simulink model "dynamicsSimulink"  (R2018a)
settings: Solver=VariableStepAuto  StartTime=0.0  StopTime=10.0  RelTol=1e-3
libraries: vehdynlibtire x4
settings Model: Creator=Raval  LastModifiedBy=Raval

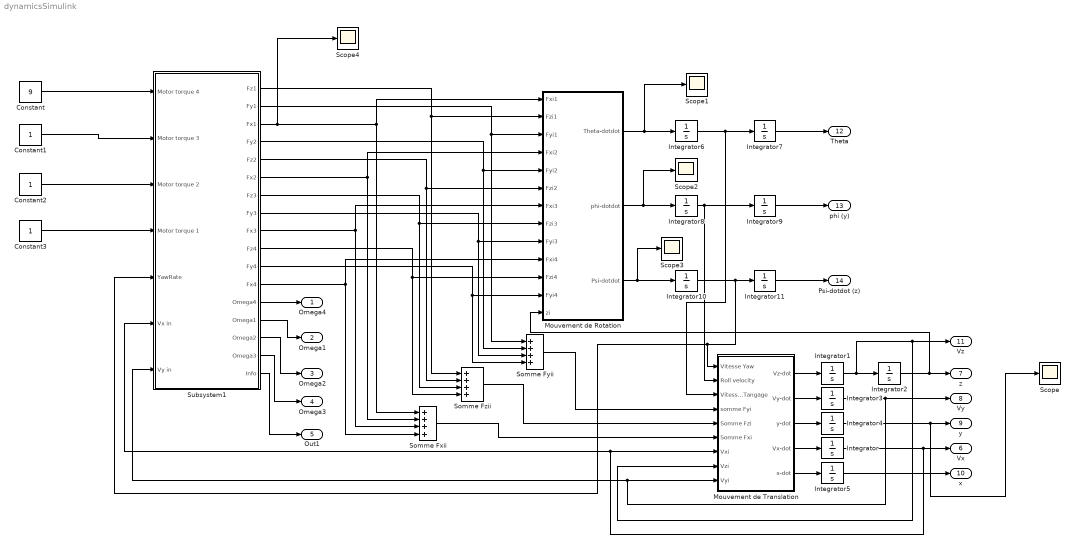
== system dynamicsSimulink ==
  Constant : Constant  Value=9
  Constant1 : Constant
  Constant2 : Constant
  Constant3 : Constant
  Integrator{,1..11} (12 alike) : Integrator
  Mouvement de Rotation : Subsystem
  Mouvement de Translation : Subsystem
  Scope{,1..4} (5 alike) : Scope
  Somme Fxii : Sum  Inputs=++++
  Somme Fyii : Sum  Inputs=++++
  Somme Fzii : Sum  Inputs=++++
  Subsystem1 : Subsystem
  Omega4 : Outport
  Omega1 : Outport  Port=2
  Omega2 : Outport  Port=3
  Omega3 : Outport  Port=4
  Out1 : Outport  Port=5
  Vx : Outport  Port=6
  z : Outport  Port=7
  Vy : Outport  Port=8
  y : Outport  Port=9
  x : Outport  Port=10
  Vz : Outport  Port=11
  Theta : Outport  Port=12
  phi (y) : Outport  Port=13
  Psi-dotdot (z) : Outport  Port=14
  wires:
  Integrator8/1 -> Mouvement de Translation/2(Roll velocity), Integrator9/1
  Integrator6/1 -> Mouvement de Translation/3(Vitesse Tangage), Integrator7/1
  Somme Fyii/1 -> Mouvement de Translation/4(somme Fyi)
  Somme Fzii/1 -> Mouvement de Translation/5(Somme Fzi)
  Somme Fxii/1 -> Mouvement de Translation/6(Somme Fxi)
  Integrator1/1 -> Mouvement de Translation/8(Vzi), Vz/1, Integrator2/1
  Mouvement de Translation/1(Vz-dot) -> Integrator1/1
  Mouvement de Translation/2(Vy-dot) -> Integrator3/1
  Mouvement de Translation/3(y-dot) -> Integrator4/1
  Mouvement de Translation/5(x-dot) -> Integrator5/1
  Subsystem1/3(Fx1) -> Scope4/1, Somme Fxii/1, Mouvement de Rotation/1(Fxi1)
  Subsystem1/1(Fz1) -> Mouvement de Rotation/2(Fzi1), Somme Fzii/1
  Subsystem1/2(Fy1) -> Mouvement de Rotation/3(Fyi1), Somme Fyii/1
  Subsystem1/6(Fx2) -> Somme Fxii/2, Mouvement de Rotation/4(Fxi2)
  Subsystem1/4(Fy2) -> Mouvement de Rotation/5(Fyi2), Somme Fyii/2
  Subsystem1/5(Fz2) -> Somme Fzii/2, Mouvement de Rotation/6(Fzi2)
  Subsystem1/9(Fx3) -> Mouvement de Rotation/7(Fxi3), Somme Fxii/3
  Subsystem1/7(Fz3) -> Somme Fzii/3, Mouvement de Rotation/8(Fzi3)
  Subsystem1/8(Fy3) -> Mouvement de Rotation/9(Fyi3), Somme Fyii/3
  Subsystem1/12(Fx4) -> Somme Fxii/4, Mouvement de Rotation/10(Fxi4)
  Subsystem1/10(Fz4) -> Somme Fzii/4, Mouvement de Rotation/11(Fzi4)
  Subsystem1/11(Fy4) -> Somme Fyii/4, Mouvement de Rotation/12(Fyi4)
  Integrator2/1 -> Mouvement de Rotation/13(zi), z/1
  Mouvement de Rotation/1(Theta-dotdot) -> Scope1/1, Integrator6/1
  Mouvement de Rotation/2(phi-dotdot) -> Scope2/1, Integrator8/1
  Mouvement de Rotation/3(Psi-dotdot) -> Scope3/1, Integrator10/1
  Constant/1 -> Subsystem1/1(Motor torque 4)
  Constant1/1 -> Subsystem1/2(Motor torque 3)
  Constant2/1 -> Subsystem1/3(Motor torque 2)
  Constant3/1 -> Subsystem1/4(Motor torque 1)
  Integrator10/1 -> Mouvement de Translation/1(Vitesse Yaw), Subsystem1/5(YawRate), Integrator11/1
  Integrator/1 -> Subsystem1/6(Vx in), Mouvement de Translation/7(Vxi), Vx/1
  Integrator3/1 -> Vy/1, Subsystem1/7(Vy in), Mouvement de Translation/9(Vyi)
  Subsystem1/13(Omega4) -> Omega4/1
  Subsystem1/14(Omega1) -> Omega1/1
  Subsystem1/15(Omega2) -> Omega2/1
  Subsystem1/16(Omega3) -> Omega3/1
  Subsystem1/17(Info) -> Out1/1
  Mouvement de Translation/4(Vx-dot) -> Integrator/1
  Integrator4/1 -> Scope/1, y/1
  Integrator5/1 -> x/1
  Integrator7/1 -> Theta/1
  Integrator9/1 -> phi (y)/1
  Integrator11/1 -> Psi-dotdot (z)/1

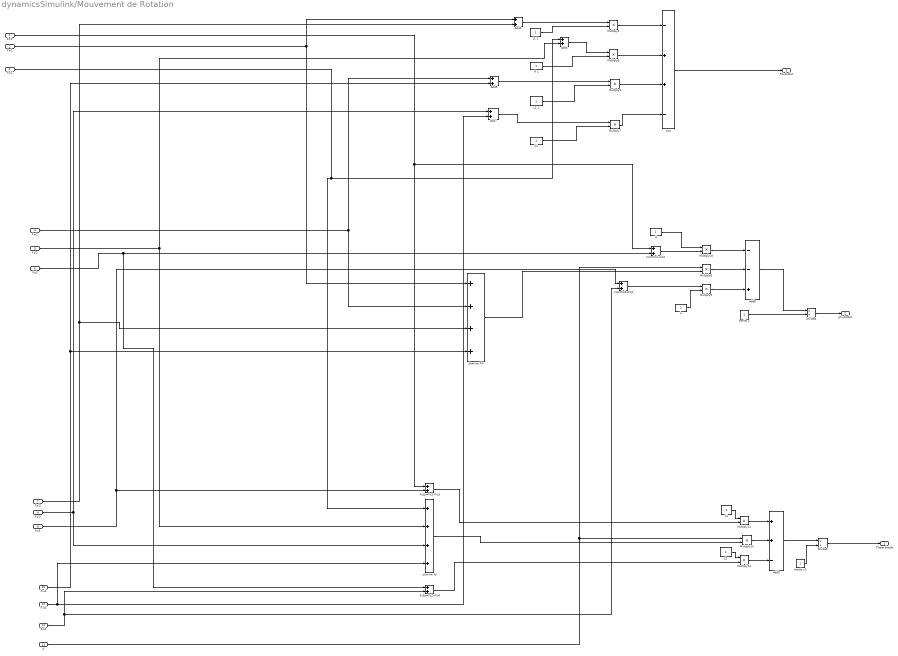
== system dynamicsSimulink/Mouvement de Rotation ==
  Fxi1 : Inport
  Fzi1 : Inport  Port=2
  Fyi1 : Inport  Port=3
  Fxi2 : Inport  Port=4
  Fyi2 : Inport  Port=5
  Fzi2 : Inport  Port=6
  Fxi3 : Inport  Port=7
  Fzi3 : Inport  Port=8
  Fyi3 : Inport  Port=9
  Fxi4 : Inport  Port=10
  Fzi4 : Inport  Port=11
  Fyi4 : Inport  Port=12
  zi : Inport  Port=13
  Add{4..7} (4 alike) : Sum
  Add8 : Sum  Inputs=--+
  Add9 : Sum  Inputs=++-
  Divide4 : Product  Inputs=*/
  Divide5 : Product  Inputs=*/
  Fs1=Fz1+Fz2 : Sum
  Fs1p=Fz1+Fz3 : Sum
  Fs2=Fz3+Fz4 : Sum
  Fs2p=Fz2+Fz4 : Sum
  Inertie x1 : Constant
  Inertie y : Constant
  "L1 " : Constant
  L1 2 : Constant
  "L2 " : Constant
  L2 1 : Constant
  Multiply{4..13} (10 alike) : Product
  Somme FXi : Sum  Inputs=++++
  Yaw : Sum  Inputs=-++-
  "lf " : Constant
  lf 1 : Constant
  lr : Constant
  lr1 : Constant
  somme fyi : Sum  Inputs=++++
  Theta-dotdot : Outport
  phi-dotdot : Outport  Port=2
  Psi-dotdot : Outport  Port=3
  wires:
  Add9/1 -> Divide5/1
  Fxi3/1 -> Somme FXi/3, Add4/2
  Yaw/1 -> Psi-dotdot/1
  Multiply9/1 -> Add8/3
  Fxi1/1 -> Add4/1, Somme FXi/1
  zi/1 -> Multiply13/1, Multiply8/1
  Fs2=Fz3+Fz4/1 -> Multiply9/1
  Fyi1/1 -> somme fyi/1, Add6/1
  Fs1p=Fz1+Fz3/1 -> Multiply11/2
  Divide4/1 -> phi-dotdot/1
  Multiply10/1 -> Add8/1
  Add8/1 -> Divide4/1
  Fyi2/1 -> somme fyi/2, Add6/2
  Fxi4/1 -> Somme FXi/4, Add5/2
  Fzi1/1 -> Fs1=Fz1+Fz2/1, Fs1p=Fz1+Fz3/1
  lr1/1 -> Multiply7/2
  Multiply8/1 -> Add8/2
  Fzi3/1 -> Fs2=Fz3+Fz4/1, Fs1p=Fz1+Fz3/2
  L2 1/1 -> Multiply5/2
  Multiply12/1 -> Add9/3
  Fyi3/1 -> somme fyi/3, Add7/1
  Add4/1 -> Multiply4/1
  Fxi2/1 -> Somme FXi/2, Add5/1
  Inertie x1/1 -> Divide5/2
  somme fyi/1 -> Multiply13/2
  lf 1/1 -> Multiply6/2
  L1 2/1 -> Multiply4/2
  Add5/1 -> Multiply5/1
  Fzi2/1 -> Fs1=Fz1+Fz2/2, Fs2p=Fz2+Fz4/1
  Divide5/1 -> Theta-dotdot/1
  Fyi4/1 -> Add7/2, somme fyi/4
  lr/1 -> Multiply9/2
  Fzi4/1 -> Fs2p=Fz2+Fz4/2, Fs2=Fz3+Fz4/2
  Inertie y/1 -> Divide4/2
  Fs1=Fz1+Fz2/1 -> Multiply10/2
  "lf "/1 -> Multiply10/1
  Multiply13/1 -> Add9/2
  Multiply6/1 -> Yaw/2
  Somme FXi/1 -> Multiply8/2
  "L1 "/1 -> Multiply11/1
  Fs2p=Fz2+Fz4/1 -> Multiply12/2
  Multiply4/1 -> Yaw/1
  Multiply7/1 -> Yaw/4
  "L2 "/1 -> Multiply12/1
  Multiply11/1 -> Add9/1
  Add6/1 -> Multiply6/1
  Add7/1 -> Multiply7/1
  Multiply5/1 -> Yaw/3

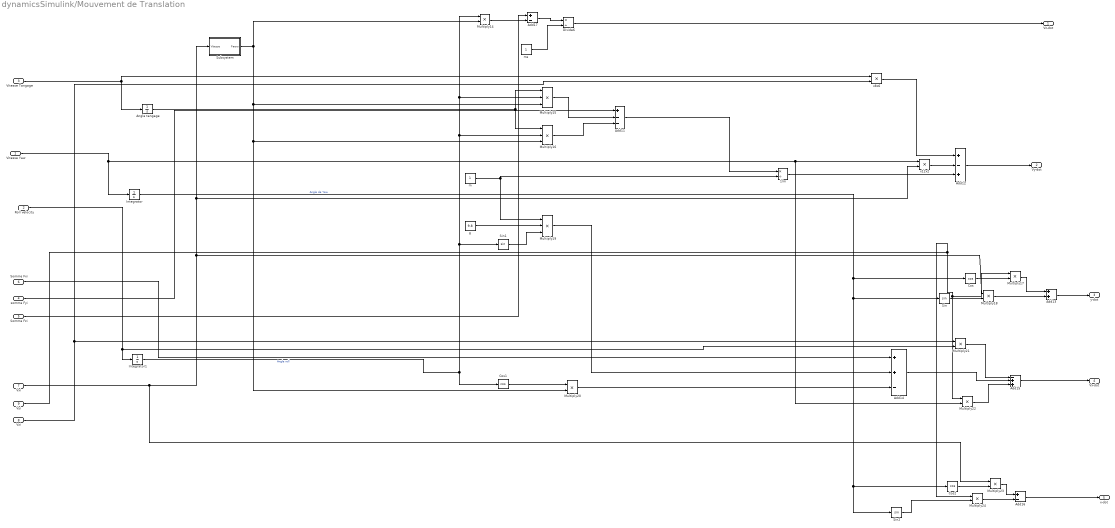
== system dynamicsSimulink/Mouvement de Translation ==
  Vitesse Yaw : Inport
  Roll velocity : Inport  Port=2
  Vitesse Tangage : Inport  Port=3
  somme Fyi : Inport  Port=4
  Somme Fzi : Inport  Port=5
  Somme Fxi : Inport  Port=6
  Vxi : Inport  Port=7
  Vzi : Inport  Port=8
  Vyi : Inport  Port=9
  1/m : Product  Inputs=*/
  Add11 : Sum  Inputs=+--
  Add12 : Sum  Inputs=+-+
  Add13 : Sum
  Add14 : Sum  Inputs=++-
  Add15 : Sum  Inputs=-++
  Add16 : Sum  Inputs=+-
  Add17 : Sum  Inputs=+-
  Angle tangage : Integrator
  Cos : Trigonometry  Operator=cos
  Cos1 : Trigonometry  Operator=cos
  Cos2 : Trigonometry  Operator=cos
  Divide6 : Product  Inputs=*/
  Integrator : Integrator
  Integrator1 : Integrator
  Multiply{14,17..18,20..24} (8 alike) : Product
  Multiply15 : Product  Inputs=3
  Multiply16 : Product  Inputs=3
  Multiply19 : Product  Inputs=3
  Sin : Trigonometry
  Sin1 : Trigonometry
  Sin2 : Trigonometry
  Subsystem : Subsystem
  g : Constant  Value=9.8
  m : Constant
  ms : Constant
  x12x2 : Product
  x8x6 : Product
  Vz-dot : Outport
  Vy-dot : Outport  Port=2
  y-dot : Outport  Port=3
  Vx-dot : Outport  Port=4
  x-dot : Outport  Port=5
  wires:
  Vzi/1 -> x8x6/2, Multiply21/1
  Vitesse Yaw/1 -> x12x2/1, Multiply22/2, Integrator/1
  Multiply23/1 -> Add16/1
  Add12/1 -> Vy-dot/1
  Roll velocity/1 -> Integrator1/1, Multiply21/2
  Vyi/1 -> Multiply24/1, Multiply17/1, Multiply22/1
  Add17/1 -> Divide6/1
  somme Fyi/1 -> Add11/1
  Multiply14/1 -> Add17/2
  Subsystem/1(Faero) -> Multiply20/2, Multiply16/3, Multiply15/3, Multiply14/2
  Add15/1 -> Vx-dot/1
  Somme Fzi/1 -> Add17/1
  Integrator/1 -> Sin2/1, Cos2/1, Sin/1, Cos/1  "Angle de Yaw"
  Multiply18/1 -> Add13/2
  Vxi/1 -> Multiply23/1, x12x2/2, Subsystem/1(Vitesse), Multiply18/1
  Integrator1/1 -> Multiply14/1, Multiply15/2, Multiply16/2, Sin1/1, Cos1/1  "Angle roll"
  Add11/1 -> 1/m/1
  Multiply19/1 -> Add14/2
  Multiply24/1 -> Add16/2
  Add14/1 -> Add15/2
  Vitesse Tangage/1 -> Angle tangage/1, x8x6/1
  Angle tangage/1 -> Multiply16/1, Multiply15/1
  Sin2/1 -> Multiply24/2
  Multiply22/1 -> Add15/3
  Add16/1 -> x-dot/1
  Somme Fxi/1 -> Add14/1
  ms/1 -> Divide6/2
  Multiply16/1 -> Add11/3
  Add13/1 -> y-dot/1
  1/m/1 -> Add12/3
  Divide6/1 -> Vz-dot/1
  Sin/1 -> Multiply18/2
  x12x2/1 -> Add12/2
  Cos/1 -> Multiply17/2
  Multiply17/1 -> Add13/1
  Cos1/1 -> Multiply20/1
  Multiply20/1 -> Add14/3
  Multiply15/1 -> Add11/2
  m/1 -> Multiply19/1, 1/m/2
  x8x6/1 -> Add12/1
  Cos2/1 -> Multiply23/2
  Multiply21/1 -> Add15/1
  Sin1/1 -> Multiply19/3
  g/1 -> Multiply19/2

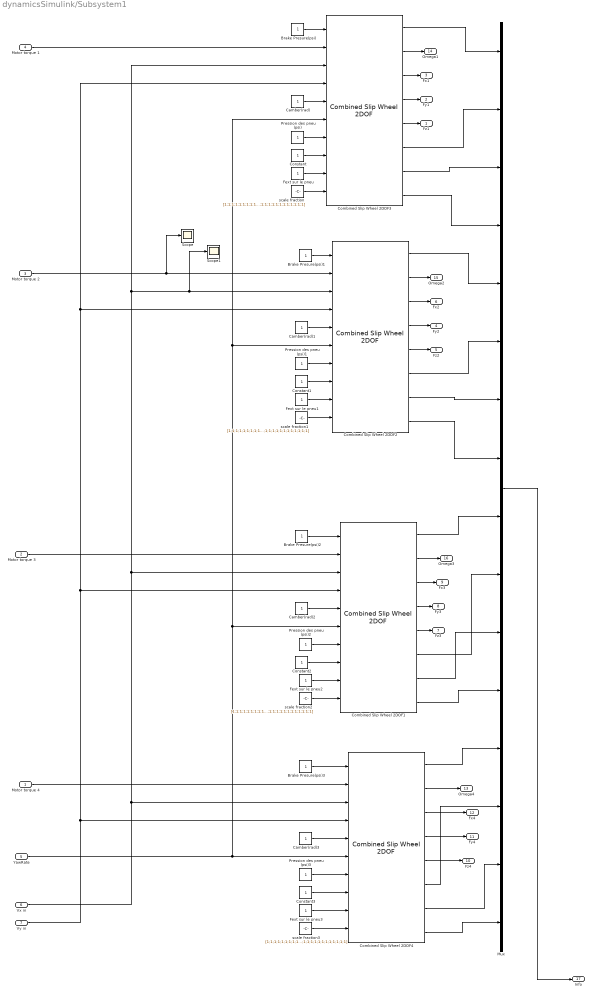
== system dynamicsSimulink/Subsystem1 ==
  Motor torque 4 : Inport
  Motor torque 3 : Inport  Port=2
  Motor torque 2 : Inport  Port=3
  Motor torque 1 : Inport  Port=4
  YawRate : Inport  Port=5
  Vx in : Inport  Port=6
  Vy in : Inport  Port=7
  Brake Presure(psi){,1..3} (4 alike) : Constant
  Camber(rad){,1..3} (4 alike) : Constant
  Combined Slip Wheel 2DOF{1..4} (4 alike) : vehdynlibtire/Combined Slip Wheel 2DOF  BrakeType=Disc  mu_static=.3  mu_kinetic=.2  disk_abore=.05  Rm=.177  num_pads=2  drum_abore=0.0508  drum_a=0.123  drum_c=0.212  drum_r=0.15  drum_theta1=0  drum_theta2=126  brake_p_bpt=[1 11.4736842105263 21.9473684210526 32.4210526315789 42.8947368421053 53.3684210526316 63.8421052631579 74.3157894736842 84.7894736842105 95.2631578947368 105.736842105263 116.210526315789 126.684210526316 137.157894736842 147.631578947368 158.105263157895 168.578947368421 179.052631578947 189.526315789474 200]  brake_n_bpt=[0 52.6315789473684 105.263157894737 157.894736842105 210.526315789474 263.157894736842 315.789473684211 368.421052631579 421.052631578947 473.684210526316 526.315789473684 578.947368421053 631.578947368421 684.210526315789 736.842105263158 789.473684210526 842.105263157895 894.736842105263 947.368421052632 1000]  f_brake_t=[43.4900602404453 42.5056030554862 41.5350898940194 40.5780454442085 39.6340111501808 38.7025443887544 37.7832176914519 36.8756180088306 35.9793460143796 35.0940154454303 34.2192524787115 33.3546951383474 32.4999927342521 31.6548053290159 30.8188032315107 29.991666515561 29.1730845621415 28.362755623661 27.5603864089927 26.765691687993;498.991217495636 487.695866636631 476.560505099801 465.579679307235 454.748127933653 444.060772460445 433.51270824929 423.099196101319 412.81565427025 402.657650900201 392.620896861006 382.701238955775 372.894653477208 363.197240090814 353.605216024701 344.114910546964 334.722759712992 325.425301366216 316.219170376863 307.10109410434;954.492374750826 932.886130217776 911.585920305583 890.581313170261 869.862244717126 849.419000532136 829.242198807128 809.322774193808 789.651962526121 770.221286354971 751.0225412433 732.047782773203 713.289314220164 694.739674852612 676.391628817892 658.238154578366 640.272434863842 622.48784710877 604.877954344734 587.436496520688;1409.99353200602 1378.07639379892 1346.61133551136 1315.58294703329 1284.9763615006 1254.77722860383 1224.97168936497 1195.5463522863 1166.48827078199 1137.78492180974 1109.42418562559 1081.39432659063 1053.68397496312 1026.28210961441 999.178041611083 972.361398609768 945.822110014692 919.550392851325 893.536738312604 867.771898937035;1865.49468926121 1823.26665738007 1781.63675071715 1740.58458089631 1700.09047828407 1660.13545667552 1620.7011799228 1581.76993037878 1543.32457903786 1505.34855726451 1467.82583000789 1430.74087040806 1394.07863570608 1357.82454437621 1321.96445440427 1286.48464264117 1251.37178516554 1216.61293859388 1182.19552228048 1148.10730135338;2320.9958465164 2268.45692096121 2216.66216592293 2165.58621475934 2115.20459506754 2065.49368474721 2016.43067048064 1967.99350847127 1920.16088729373 1872.91219271928 1826.22747439018 1780.08741422549 1734.47329644903 1689.36697913801 1644.75086719747 1600.60788667257 1556.92146031639 1513.67548433643 1470.85430624835 1428.44270376973;2776.49700377159 2713.64718454235 2651.68758112871 2590.58784862237 2530.31871185102 2470.8519128189 2412.16016103848 2354.21708656376 2296.9971955496 2240.47582817405 2184.62911877248 2129.43395804292 2074.86795719199 2020.9094138998 1967.53727999066 1914.73113070398 1862.47113546724 1810.73803007899 1759.51309021622 1708.77810618608;3231.99816102678 3158.8374481235 3086.71299633449 3015.58948248539 2945.43282863449 2876.21014089059 2807.88965159632 2740.44066465625 2673.83350380547 2608.03946362882 2543.03076315477 2478.78050186034 2415.26261793494 2352.4518486616 2290.32369278385 2228.85437473538 2168.02081061809 2107.80057582154 2048.17187418409 1989.11350860242;3687.49931828197 3604.02771170464 3521.73841154027 3440.59111634842 3360.54694541796 3281.56836896228 3203.61914215416 3126.66424274874 3050.66981206134 2975.60309908359 2901.43240753707 2828.12704567777 2755.6572786779 2683.9942834234 2613.11010557704 2542.97761876678 2473.57048576894 2404.8631215641 2336.83065815196 2269.44891101877;4143.00047553716 4049.21797528579 3956.76382674606 3865.59275021144 3775.66106220143 3686.92659703397 3599.34863271199 3512.88782084123 3427.50612031721 3343.16673453836 3259.83405191936 3177.4735894952 3096.05193942085 3015.5367181852 2935.89651837023 2857.10086279818 2779.12016091979 2701.92566730665 2625.48944211983 2549.78431343512;4598.50163279235 4494.40823886693 4391.78924195184 4290.59438407447 4190.77517898491 4092.28482510566 3995.07812326983 3899.11139893372 3804.34242857308 3710.73036999313 3618.23569630166 3526.82013331263 3436.44660016381 3347.079152947 3258.68293116342 3171.22410682959 3084.66983607064 2998.98821304921 2914.1482260877 2830.11971585147;5054.00279004754 4939.59850244808 4826.81465715762 4715.59601793749 4605.88929576838 4497.64305317735 4390.80761382767 4285.3349770262 4181.17873682896 4078.2940054479 3976.63734068395 3876.16667713006 3776.84126090677 3678.62158770879 3581.46934395661 3485.34735086099 ...(+2764 chars)]  tireParamSet=vdynPassCar.mat  plySteer=off  turnslip=off  PRESMAX=1003118.65547859  PRESMIN=9982.11955979412  FZMAX=10000  FZMIN=100  VXLOW=0.1  KPUMAX=1.48764378595932  KPUMIN=-1.48007456759542  ALPMAX=1.47424202250808  ALPMIN=-1.50806269049027  CAMMAX=0.173142086627737  CAMMIN=-0.173348165334087  LONGVL=16.7  omegao=0  br=1e-3  UNLOADED_RADIUS=0.309384029954441  NOMPRES=224006.174898101  FNOMIN=4024.75203401849  WIDTH=0.209045013245853  MASS=9.46491996974568  IYY=0.740633832792491  GRAVITY=-9.81  zo=0  zdoto=0  BREFF=8.25094594147963  DREFF=0.260468730454265  FREFF=0.0735298544471851  Q_RE0=1.00866439868088  Q_V1=0.000760413786224011  Q_V2=0.0463384792019201  Q_FZ1=0  Q_FZ2=15.6870832810226  Q_FZ3=0  Q_FCX=0.138643970247602  Q_FCY=0.10843499565426  Q_FCY2=-0.465763352339538  PFZ1=0.69958166705601  VERTICAL_STIFFNESS=207885.061134007  VERTICAL_DAMPING=494.649255786991  LONGITUDINAL_STIFFNESS=388714.175879854  LATERAL_STIFFNESS=157087.404633332  PCFX1=0.18539229191199  PCFX2=0  PCFX3=0  PCFY1=0.163183345037677  PCFY2=0  PCFY3=0.249094918231954  Q_RA1=0.675942571700787  Q_RA2=0.73800463546164  Q_RB1=1.04487486456705  Q_RB2=-1.191763806629  PCX1=1.58523057950359  PDX1=1.0239116238178  PDX2=-0.0842405110022724  PDX3=0  PEX1=0.110312777158455  PEX2=0.313468516038146  PEX3=0  PEX4=0.0016060905760045  PKX1=21.3872544684023  PKX2=14.0006541873175  PKX3=-0.405326109653452  PHX1=0.000212599305364818  PHX2=0.00115950515263055  PVX1=1.59236164471432e-05  PVX2=0.000104321112127671  PPX1=-0.349461321276586  PPX2=0.387840040616429  PPX3=-0.0969947336569324  PPX4=0.0632271859795801  RBX1=12.7633329850276  RBX2=9.5787123658471  RBX3=0  RCX1=1.02796280922059  REX1=-0.45202516851367  REX2=-0.47304886171176  RHX1=0.000233272373115809  QSX1=-0.00788307788961443  QSX2=0.954629515459396  QSX3=0.0155855777667025  QSX4=0.125904607142414  QSX5=1.01110069703963  QSX6=20.1938577118433  QSX7=0.310818120717083  QSX8=-0.0430823751139655  QSX9=0.636494404888216  QSX10=0.142438060591663  QSX11=0.346766530036373  QSX12=0  QSX13=0  QSX14=0  PPMX1=0  PCY1=1.34299950037631  PDY1=0.878267729082195  PDY2=-0.0644597923147385  PDY3=0  PEY1=-0.809776534470972  PEY2=-0.600180598867198  PEY3=0.0991732552633487  PEY4=-6.5577974035573  PEY5=0  PKY1=-15.5714726518315  PKY2=1.73126522291751  PKY3=0.365349873517229  PKY4=1.98176755955416  PKY5=0  PKY6=-0.884005199550313  PKY7=-0.237259727611847  PHY1=-0.00183370557235628  PHY2=0.00346401302716671  PVY1=-0.00675427560163264  PVY2=0.036379218103843  PVY3=-0.163543984089166  PVY4=-0.491003349625726  PPY1=-0.62059646553185  PPY2=-0.0647824842338686  PPY3=-0.164648843290686  PPY4=0.283193909060098  PPY5=0  RBY1=10.7588809173639  RBY2=7.70420065295029  RBY3=3.40283755070691e-06  RBY4=0  RCY1=1.06691874059059  REY1=0.308244924574305  REY2=7.48775032604508e-06  RHY1=0.0118479204960415  RHY2=7.63650177161071e-06  RVY1=0.0560024425050078  RVY2=7.48487127056197e-06  RVY3=0  RVY4=98.4047026517149  RVY5=2.02759273900054  RVY6=15.7623064923347  QSY1=0.00699077564863536  QSY2=0  QSY3=0.00153535478298811  QSY4=8.55710322455322e-05  QSY5=0  QSY6=0  QSY7=0.89443879773793  QSY8=-0.403227641260894  QBZ1=11.666656027484  QBZ2=-1.30355438574485  QBZ3=0  QBZ4=0.177918305399071  QBZ5=-0.162481135068033  QBZ6=0  QBZ9=30.1445534682089  QBZ10=0  QCZ1=1.29026978207574  QDZ1=0.0886972644991399  QDZ2=-0.0058634820161856  QDZ3=0.3805597481383  QDZ4=0  QDZ6=0.00160914918118959  QDZ7=-0.00211036330862154  QDZ8=-0.13921904912557  QDZ9=0.00816585550028243  QDZ10=0  QDZ11=0  QEZ1=-2.19802254534746  QEZ2=1.01850535789165  QEZ3=0  QEZ4=0.278379679112054  QEZ5=-0.548414722765386  QHZ1=0.00148361198869669  QHZ2=0.00202017567585904  QHZ3=0.240316641332066  QHZ4=-0.210114035738085  PPZ1=-0.443927982388615  PPZ2=0  SSZ1=0.00914999585397887  SSZ2=0.0389830656052735  SSZ3=0  SSZ4=0  PDXP1=0.396718274678791  PDXP2=0  PDXP3=0  PKYP1=1.00587060633573  PDYP1=0.40483048923438  PDYP2=0  PDYP3=0  PDYP4=0  PHYP1=0.992731942067188  PHYP2=0.150352945499914  PHYP3=0  PHYP4=-3.98988682633674  PECP1=0.502379254513503  PECP2=0  QDTP1=10.0178654287947  QCRP1=0.200627747200702  QCRP2=0.0995735881599772  QBRP1=0.0997107127960717  QDRP1=1.01432910167423  QDRP2=0  aMode=2
      settings: SourceProductName=Vehicle Dynamics Blockset  SourceProductBaseCode=VE
  Constant{,1..3} (4 alike) : Constant
  Fext sur le pneu{,1..3} (4 alike) : Constant
  Mux : Mux  Inputs=16
  Pression des pneu (psi){,1..3} (4 alike) : Constant
  Scope : Scope
  Scope1 : Scope
  scale fraction{,1..3} (4 alike) : Constant  Value=[1;1;1;1;1;1;1;1;1;1;1;1;1;1;1;1;1;1;1;1;1;1;1;1;1;1;1]  VectorParams1D=off
  Fz1 : Outport
  Fy1 : Outport  Port=2
  Fx1 : Outport  Port=3
  Fy2 : Outport  Port=4
  Fz2 : Outport  Port=5
  Fx2 : Outport  Port=6
  Fz3 : Outport  Port=7
  Fy3 : Outport  Port=8
  Fx3 : Outport  Port=9
  Fz4 : Outport  Port=10
  Fy4 : Outport  Port=11
  Fx4 : Outport  Port=12
  Omega4 : Outport  Port=13
  Omega1 : Outport  Port=14
  Omega2 : Outport  Port=15
  Omega3 : Outport  Port=16
  Info : Outport  Port=17
  wires:
  Combined Slip Wheel 2DOF1/1 -> Mux/9
  Vx in/1 -> Combined Slip Wheel 2DOF3/3, Scope1/1, Combined Slip Wheel 2DOF2/3, Combined Slip Wheel 2DOF1/3, Combined Slip Wheel 2DOF4/3
  Camber(rad)1/1 -> Combined Slip Wheel 2DOF2/5
  Combined Slip Wheel 2DOF3/1 -> Mux/1
  YawRate/1 -> Combined Slip Wheel 2DOF3/6, Combined Slip Wheel 2DOF2/6, Combined Slip Wheel 2DOF1/6, Combined Slip Wheel 2DOF4/6
  Combined Slip Wheel 2DOF3/3 -> Fx1/1
  Combined Slip Wheel 2DOF2/1 -> Mux/5
  Combined Slip Wheel 2DOF3/4 -> Fy1/1
  Combined Slip Wheel 2DOF4/1 -> Mux/13
  Vy in/1 -> Combined Slip Wheel 2DOF3/4, Combined Slip Wheel 2DOF2/4, Combined Slip Wheel 2DOF1/4, Combined Slip Wheel 2DOF4/4
  Combined Slip Wheel 2DOF2/5 -> Fz2/1
  Combined Slip Wheel 2DOF3/8 -> Mux/4
  scale fraction/1 -> Combined Slip Wheel 2DOF3/10
  Combined Slip Wheel 2DOF4/6 -> Mux/14
  Combined Slip Wheel 2DOF1/8 -> Mux/12
  Combined Slip Wheel 2DOF2/8 -> Mux/8
  Combined Slip Wheel 2DOF1/3 -> Fx3/1
  Motor torque 1/1 -> Combined Slip Wheel 2DOF3/2
  Combined Slip Wheel 2DOF4/5 -> Fz4/1
  Fext sur le pneu1/1 -> Combined Slip Wheel 2DOF2/9
  Combined Slip Wheel 2DOF3/2 -> Omega1/1
  Camber(rad)/1 -> Combined Slip Wheel 2DOF3/5
  Combined Slip Wheel 2DOF4/7 -> Mux/15
  Brake Presure(psi)2/1 -> Combined Slip Wheel 2DOF1/1
  Constant3/1 -> Combined Slip Wheel 2DOF4/8
  Combined Slip Wheel 2DOF2/2 -> Omega2/1
  Fext sur le pneu3/1 -> Combined Slip Wheel 2DOF4/9
  Fext sur le pneu/1 -> Combined Slip Wheel 2DOF3/9
  Combined Slip Wheel 2DOF3/7 -> Mux/3
  Constant1/1 -> Combined Slip Wheel 2DOF2/8
  Combined Slip Wheel 2DOF3/6 -> Mux/2
  Combined Slip Wheel 2DOF4/4 -> Fy4/1
  Combined Slip Wheel 2DOF2/6 -> Mux/6
  scale fraction2/1 -> Combined Slip Wheel 2DOF1/10
  Combined Slip Wheel 2DOF2/7 -> Mux/7
  Combined Slip Wheel 2DOF1/6 -> Mux/10
  Combined Slip Wheel 2DOF2/3 -> Fx2/1
  Mux/1 -> Info/1
  Fext sur le pneu2/1 -> Combined Slip Wheel 2DOF1/9
  scale fraction1/1 -> Combined Slip Wheel 2DOF2/10
  Combined Slip Wheel 2DOF1/2 -> Omega3/1
  Combined Slip Wheel 2DOF4/8 -> Mux/16
  Combined Slip Wheel 2DOF3/5 -> Fz1/1
  Combined Slip Wheel 2DOF1/7 -> Mux/11
  Motor torque 4/1 -> Combined Slip Wheel 2DOF4/2
  Camber(rad)3/1 -> Combined Slip Wheel 2DOF4/5
  Pression des pneu (psi)1/1 -> Combined Slip Wheel 2DOF2/7
  Combined Slip Wheel 2DOF1/4 -> Fy3/1
  Brake Presure(psi)1/1 -> Combined Slip Wheel 2DOF2/1
  Constant/1 -> Combined Slip Wheel 2DOF3/8
  Combined Slip Wheel 2DOF1/5 -> Fz3/1
  Pression des pneu (psi)2/1 -> Combined Slip Wheel 2DOF1/7
  scale fraction3/1 -> Combined Slip Wheel 2DOF4/10
  Combined Slip Wheel 2DOF4/3 -> Fx4/1
  Brake Presure(psi)/1 -> Combined Slip Wheel 2DOF3/1
  Pression des pneu (psi)/1 -> Combined Slip Wheel 2DOF3/7
  Camber(rad)2/1 -> Combined Slip Wheel 2DOF1/5
  Constant2/1 -> Combined Slip Wheel 2DOF1/8
  Brake Presure(psi)3/1 -> Combined Slip Wheel 2DOF4/1
  Motor torque 2/1 -> Scope/1, Combined Slip Wheel 2DOF2/2
  Motor torque 3/1 -> Combined Slip Wheel 2DOF1/2
  Pression des pneu (psi)3/1 -> Combined Slip Wheel 2DOF4/7
  Combined Slip Wheel 2DOF2/4 -> Fy2/1
  Combined Slip Wheel 2DOF4/2 -> Omega4/1

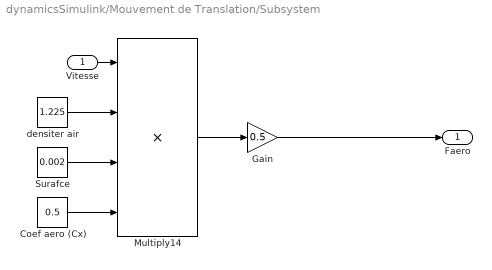
== system dynamicsSimulink/Mouvement de Translation/Subsystem ==
  Vitesse : Inport
  Coef aero (Cx) : Constant  Value=0.5
  Gain : Gain  Gain=0.5
  Multiply14 : Product  Inputs=4
  Surafce : Constant  Value=0.002
  densiter air : Constant  Value=1.225
  Faero : Outport
  wires:
  Vitesse/1 -> Multiply14/1
  densiter air/1 -> Multiply14/2
  Surafce/1 -> Multiply14/3
  Coef aero (Cx)/1 -> Multiply14/4
  Multiply14/1 -> Gain/1
  Gain/1 -> Faero/1
